simulink model "Benchmark19ARP24"  (R2023b)
settings: Solver=VariableStepAuto  StartTime=0.0  StopTime=20  RelTol=1e-3
libraries: simulink x1
settings Model: Creator=Joseph Mockler  LastModifiedBy=Joseph Mockler

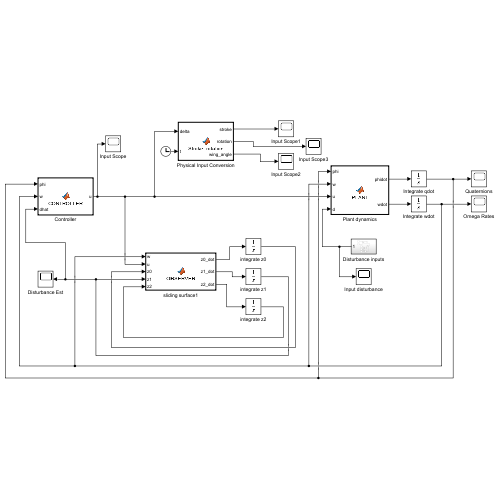
[thumbnail: Simulink's stored preview of the top-level diagram]
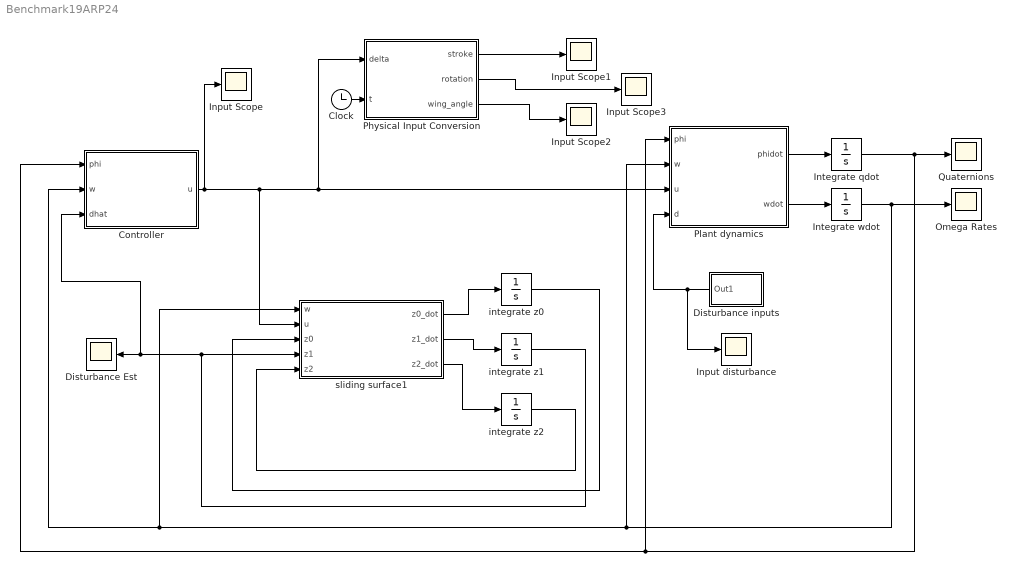
== system Benchmark19ARP24 ==
  Clock : Clock
  Controller : MATLAB Function  TreatAsAtomicUnit=on
  Disturbance Est : Scope
  Disturbance inputs : Subsystem
  Input Scope{,1..3} (4 alike) : Scope
  Input disturbance : Scope
  Integrate qdot : Integrator  InitialCondition=[10*(pi/180), 5*(pi/180), 15*(pi/180),]'
  Integrate wdot : Integrator
  Omega Rates : Scope
  Physical Input Conversion : MATLAB Function  TreatAsAtomicUnit=on
  Plant dynamics : MATLAB Function  TreatAsAtomicUnit=on
  Quaternions : Scope
  integrate z0 : Integrator
  integrate z1 : Integrator
  integrate z2 : Integrator
  sliding surface1 : MATLAB Function  TreatAsAtomicUnit=on
  wires:
  Plant dynamics/1(phidot) -> Integrate qdot/1
  Plant dynamics/2(wdot) -> Integrate wdot/1
  sliding surface1/1(z0_dot) -> integrate z0/1
  Integrate wdot/1 -> Omega Rates/1, Controller/2(w), sliding surface1/1(w), Plant dynamics/2(w)
  sliding surface1/2(z1_dot) -> integrate z1/1
  sliding surface1/3(z2_dot) -> integrate z2/1
  Integrate qdot/1 -> Quaternions/1, Controller/1(phi), Plant dynamics/1(phi)
  integrate z2/1 -> sliding surface1/5(z2)
  integrate z0/1 -> sliding surface1/3(z0)
  integrate z1/1 -> Controller/3(dhat), Disturbance Est/1, sliding surface1/4(z1)
  Controller/1(u) -> Plant dynamics/3(u), Physical Input Conversion/1(delta), sliding surface1/2(u), Input Scope/1
  Physical Input Conversion/1(stroke) -> Input Scope1/1
  Clock/1 -> Physical Input Conversion/2(t)
  Physical Input Conversion/3(wing_angle) -> Input Scope2/1
  Physical Input Conversion/2(rotation) -> Input Scope3/1
  Disturbance inputs/1(Out1) -> Input disturbance/1, Plant dynamics/4(d)

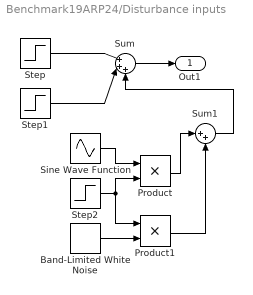
== system Benchmark19ARP24/Disturbance inputs ==
  Band-Limited White Noise : simulink/Sources/Band-Limited White Noise  Cov=[0.1]  Ts=0.1  seed=[23341]
  Product : Product
  Product1 : Product
  Sine Wave Function : Sin  Amplitude=[3, 0.2, 0.5]'  Bias=[2, -1, 1]';  Frequency=[3*pi, 2*pi, 1]';  SampleTime=0
  Step : Step  Time=5  Before=[0, 0, 0]'  After=3.*[200, -200, 100]'  SampleTime=0
  Step1 : Step  Time=10  Before=[0, 0, 0]'  After=-3.*[200, -200, 100]'  SampleTime=0
  Step2 : Step  Time=10  Before=[0, 0, 0]'  After=[10, 10, 10]';  SampleTime=0
  Sum : Sum  Inputs=|+++
  Sum1 : Sum  Inputs=|++
  Out1 : Outport
  wires:
  Sum1/1 -> Sum/3
  Product/1 -> Sum1/1
  Product1/1 -> Sum1/2
  Band-Limited White Noise/1 -> Product1/2
  Step1/1 -> Sum/2
  Sine Wave Function/1 -> Product/1
  Step2/1 -> Product1/1, Product/2
  Step/1 -> Sum/1
  Sum/1 -> Out1/1

== matlab function Benchmark19ARP24/Controller ==
  data: phi input; w input; u output; dhat input
function u = CONTROLLER(phi, w, dhat)

u = [0;0;0];

%C1 = (Ixz)/(Ixx*Izz-Ixz^2);
%C2 = (Ixx)/(Ixx*Izz-Ixz^2);
%C3 = 1/Iyy;
%C4 = (Izz)/(Ixx*Izz-Ixz^2);


%A = [C4*Lp, 0, C1*Nr;
%    0, C3*Mq, 0;
%    Cq*Lp, 0, C2*Nr];
%B = [C4*Ldp, C1*Ndb, 0;
%    0, 0, C3*Mp;
%    C1*Ldp, C2*Ndb, 0];

A = [-15.20, 0, -19.31;
    0, -2.61, 0;
    -8.13, 0, -43.18];

B = [4275.35, 2860.64, 0;
    0, 0, 3590.66;
    2288.51, 6397.42, 0];

phiR = phi(1);
phiP = phi(2);
phiY = phi(3);

T = [1, sin(phiR)*tan(phiP), cos(phiR)*tan(phiP);
    0, cos(phiR), -sin(phiR);
    0, sin(phiR)*sec(phiP), cos(phiR)*sec(phiP)];


G = 20*eye(3);
k1 = 20;
k2 = 500;
s = w + G*phi;


u = -inv(B)*((A*w + 0.5*G*T*w) + dhat + k1*s + k2*sat(s));
%u = -inv(B)*((A*w + 0.5*G*T*w) + dhat + k1*s + k2*s_sigma);

function y = sat(x)
  eps = 0.20;
  y = zeros(numel(x), 1);
  for i=1:numel(x)
    if abs(x(i)/eps)<=1
        y(i) = x(i)/eps;
    else
        y(i) = sign(x(i)/eps);
    end
  end
end

end

== matlab function Benchmark19ARP24/Plant dynamics ==
  data: phi input; w input; phidot output; u input; d input; wdot output
function [phidot, wdot] = PLANT(phi, w, u, d)

phidot = [0;0;0];
wdot = [0;0;0];

%C1 = (Ixz)/(Ixx*Izz-Ixz^2);
%C2 = (Ixx)/(Ixx*Izz-Ixz^2);
%C3 = 1/Iyy;
%C4 = (Izz)/(Ixx*Izz-Ixz^2);

phiR = phi(1);
phiP = phi(2);
phiY = phi(3);

%A = [C4*Lp, 0, C1*Nr;
%    0, C3*Mq, 0;
%    Cq*Lp, 0, C2*Nr];
%B = [C4*Ldp, C1*Ndb, 0;
%    0, 0, C3*Mp;
%    C1*Ldp, C2*Ndb, 0];

A = [-15.20, 0, -19.31;
    0, -2.61, 0;
    -8.13, 0, -43.18];

B = [4275.35, 2860.64, 0;
    0, 0, 3590.66;
    2288.51, 6397.42, 0];

T = [1, sin(phiR)*tan(phiP), cos(phiR)*tan(phiP);
    0, cos(phiR), -sin(phiR);
    0, sin(phiR)*sec(phiP), cos(phiR)*sec(phiP)];

phidot = T*w;
wdot = A*w + B*u + d;

== matlab function Benchmark19ARP24/Physical Input Conversion ==
  data: delta input; stroke output; rotation output; wing_angle output; t input
function [stroke, rotation, wing_angle] = Stroke_rotation(delta, t)

f = 60; %Hz

cap_phi_L = 120-delta(1)*(180/pi);
cap_phi_R = 120+delta(1)*(180/pi);

cap_psi_L = 120-delta(2)*(180/pi);
cap_psi_R = 120+delta(2)*(180/pi);

% Vectors are left, right

% Stroke plane
phi_L = (cap_phi_L/2)*sin(2*pi*f*t);
phi_R = (cap_phi_R/2)*sin(2*pi*f*t);
stroke = [phi_L, phi_R]';

% Rotation
psi_L = (cap_psi_L/2)*sin(2*pi*f*t);
psi_R = (cap_psi_R/2)*sin(2*pi*f*t);
rotation = [psi_L, psi_R]';

% Wing Angle
wing_angle = [delta(3)*(180/pi), -delta(3)*(180/pi)]';

end

== matlab function Benchmark19ARP24/sliding surface1 ==
  data: w input; u input; z0 input; z1 input; z0_dot output; z2 input; z1_dot output; z2_dot output
function [z0_dot, z1_dot, z2_dot] = OBSERVER(w, u, z0, z1, z2)

z0_dot = [0;0;0];
z1_dot = [0;0;0];
z2_dot = [0;0;0];

A = [-15.20, 0, -19.31;
    0, -2.61, 0;
    -8.13, 0, -43.18];

B = [4275.35, 2860.64, 0;
    0, 0, 3590.66;
    2288.51, 6397.42, 0];

L = 1000;
L0 = L^(1/3)*eye(3);
L1 = L^(2/3)*eye(3);
L2 = L^(0)*eye(3);

lambda0 = 3;
lambda1 = 1.5*sqrt(3);
lambda2 = 1.1;
n = 2;

error = z0-w;

sigma0 = [abs(error(1))^(2/3)*sign(error(1));
        abs(error(2))^(2/3)*sign(error(2))
        abs(error(3))^(2/3)*sign(error(3))];

sigma1 = [abs(error(1))^(1/3)*sign(error(1));
        abs(error(2))^(1/3)*sign(error(2))
        abs(error(3))^(1/3)*sign(error(3))];

sigma2 = [abs(error(1))^(0)*sign(error(1));
        abs(error(2))^(0)*sign(error(2))
        abs(error(3))^(0)*sign(error(3))];

z0_dot = -lambda2*L0*(sigma0) + A*w + B*u + z1;
z1_dot = -lambda1*L1*(sigma1) + z2;
z2_dot = -lambda0*L2*(sigma2);
